simulink model "com_FT60"  (R2024b)
settings: Solver=FixedStepAuto  StartTime=0.0  StopTime=60  RelTol=1e-3
values from neighbouring files (symbols this model uses):
  node = scgtnodestruct(node)    [initializeSCRAMNetGT.m]    (also in initializeSCRAMNetGT_com.m)
libraries: speedgoatlib_IO901_IO902 x3, slrealtimesharedmemorylib x2
settings Model: Creator=estructuras  LastModifiedBy=estructuras
settings SolverCC: ConcurrentTasks=on  PositivePriorityOrder=on
settings OptimizationCC: BlockReduction=off  OptimizeBlockIOStorage=off
settings DebuggingCC: TasksWithSamePriorityMsg=none
settings HardwareCC: ProdBitPerLong=64  ProdLongLongMode=on  ProdHWDeviceType=Intel->x86-64 (Linux 64)
settings RTWCC: Description=Speedgoat Real-Time Target Machine  SystemTargetFile=speedgoat.tlc  TemplateMakefile=slrealtime_default_tmf  Toolchain=Simulink Real-Time Toolchain  BuildConfiguration=Faster Runs  CodeExecutionProfiling=on  TargetLang=C++
settings SimulinkRealTimeTargetCC: InstructionSetFMA=off  LogToMDFFile=off

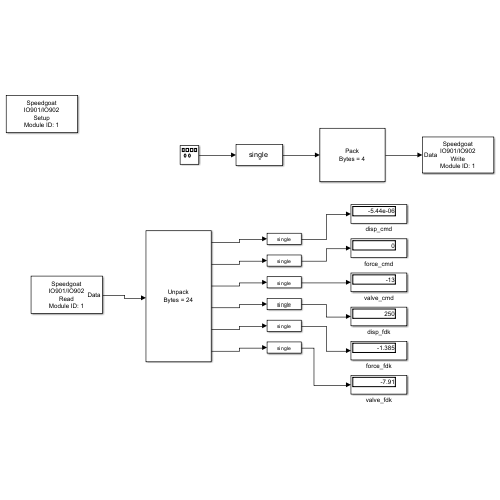
[thumbnail: Simulink's stored preview of the top-level diagram]
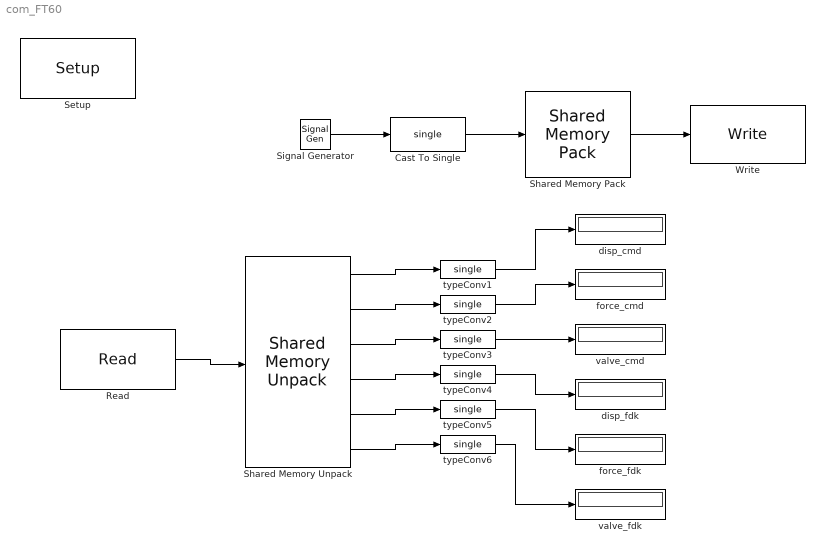
== system com_FT60 ==
  Cast To Single : DataTypeConversion  OutDataTypeStr=single  SaturateOnIntegerOverflow=off  RndMeth=Floor
  "Read " : speedgoatlib_IO901_IO902/Read   id=1  partition=node.Partitions(8:13)  ts=1  pci=-1
      settings: SourceProductName=IO901 IO902
  "Setup " : speedgoatlib_IO901_IO902/Setup   id=1  node=node  pci=-1
      settings: SourceProductName=IO901 IO902
  Shared Memory Pack : slrealtimesharedmemorylib/Shared Memory Pack  partition=node.Partitions(3)
  Shared Memory Unpack : slrealtimesharedmemorylib/Shared Memory Unpack  partition=node.Partitions(8:13)
  Signal Generator : SignalGenerator  Amplitude=50  Frequency=0.1
  "Write " : speedgoatlib_IO901_IO902/Write   id=1  partition=node.Partitions(3)  ts=0.001  pci=-1
      settings: SourceProductName=IO901 IO902
  disp_cmd : Display
      settings: Decimation=3
  disp_fdk : Display
      settings: Decimation=3
  force_cmd : Display
      settings: Decimation=3
  force_fdk : Display
      settings: Decimation=3
  typeConv{1..6} (6 alike) : DataTypeConversion  OutDataTypeStr=single
  valve_cmd : Display
      settings: Decimation=3
  valve_fdk : Display
      settings: Decimation=3
  wires:
  Cast To Single/1 -> Shared Memory Pack/1
  Shared Memory Pack/1 -> "Write "/1
  Shared Memory Unpack/1 -> typeConv1/1
  "Read "/1 -> Shared Memory Unpack/1
  Signal Generator/1 -> Cast To Single/1
  typeConv1/1 -> disp_cmd/1
  typeConv2/1 -> force_cmd/1
  typeConv3/1 -> valve_cmd/1
  typeConv4/1 -> disp_fdk/1
  typeConv5/1 -> force_fdk/1
  typeConv6/1 -> valve_fdk/1
  Shared Memory Unpack/2 -> typeConv2/1
  Shared Memory Unpack/3 -> typeConv3/1
  Shared Memory Unpack/4 -> typeConv4/1
  Shared Memory Unpack/5 -> typeConv5/1
  Shared Memory Unpack/6 -> typeConv6/1
